simulink model "sys"  (R2020b)
settings: Solver=VariableStepAuto  StartTime=0.0  StopTime=10  RelTol=1e-3
values from neighbouring files (symbols this model uses):
  A = - 1 / (epsilon * Td)    (= -10)    [script.m]
  B = [ 1/(epsilon * Td) 0 ]    [script.m]
  C = kd / epsilon    (= 0.0001)    [script.m]
  D = [ -k-kd/epsilon kr ]    [script.m]
  stateBar = [ hBar; qBar; NBar ]    [script.m]
  uBar = 0    [script.m]
libraries: simulink x1
settings Model: Creator=thoma  LastModifiedBy=thoma

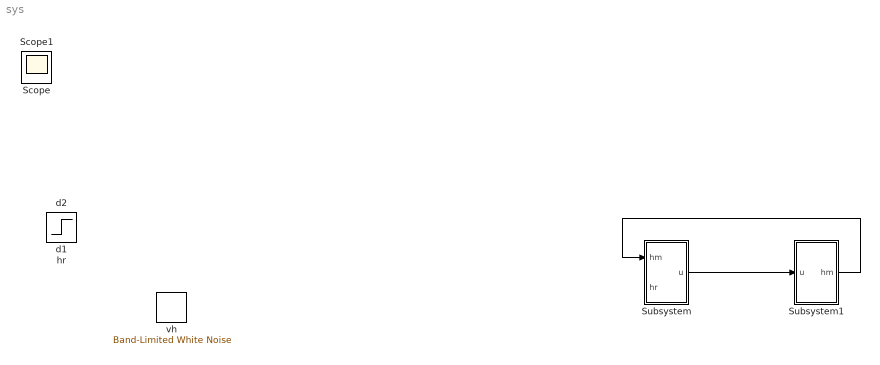
== system sys ==
  Subsystem : Subsystem
  Subsystem1 : Subsystem
  Scope : Scope
  Scope1 : Scope
  d1 : Step  IOType=siggen  After=0.2  SampleTime=0
  d2 : Step  IOType=siggen  Time=4  After=-1  SampleTime=0
  hr : Step  IOType=siggen  After=0  SampleTime=0
  vh : simulink/Sources/Band-Limited White Noise  IOType=siggen  Cov=1e-6  Ts=1e-2  seed=10
  wires:
  Subsystem/1(u) -> Subsystem1/1(u)
  Subsystem1/1(hm) -> Subsystem/1(hm)

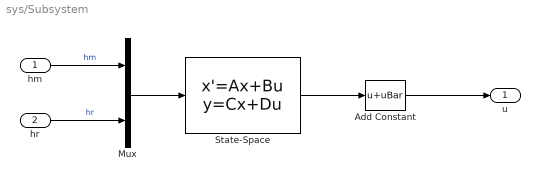
== system sys/Subsystem ==
  hm : Inport
  hr : Inport  Port=2
  Add Constant : Bias  Bias=uBar
  Mux : Mux  Inputs=2
  State-Space : StateSpace  A=A  B=B  C=C  D=D  InitialCondition=0
  u : Outport
  wires:
  Mux/1 -> State-Space/1
  State-Space/1 -> Add Constant/1
  Add Constant/1 -> u/1
  hm/1 -> Mux/1  "hm"
  hr/1 -> Mux/2  "hr"

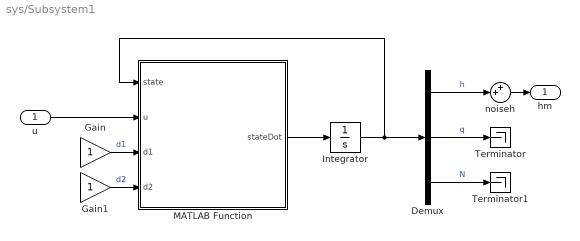
== system sys/Subsystem1 ==
  u : Inport
  Demux : Demux  Outputs=3
  Gain : Gain
  Gain1 : Gain
  Integrator : Integrator  InitialCondition=stateBar
  MATLAB Function : MATLAB Function  TreatAsAtomicUnit=on
  Terminator : Terminator
  Terminator1 : Terminator
  noiseh : Sum  Inputs=++|
  hm : Outport
  wires:
  Demux/3 -> Terminator1/1  "N"
  Demux/2 -> Terminator/1  "q"
  noiseh/1 -> hm/1
  Integrator/1 -> MATLAB Function/1(state), Demux/1
  Demux/1 -> noiseh/2  "h"
  MATLAB Function/1(stateDot) -> Integrator/1
  u/1 -> MATLAB Function/2(u)
  Gain/1 -> MATLAB Function/3(d1)  "d1"
  Gain1/1 -> MATLAB Function/4(d2)  "d2"

== matlab function sys/Subsystem1/MATLAB Function ==
  data: state input; u input; stateDot output; d1 input; d2 input
function stateDot = fcn(state, u, d1, d2)
h = state(1);
q = state(2);
N = state(3);

a = 1.0;
b = 2.5;
c = 0.1;
hBar = 0;
NBar = a/b;

hDot = q;
qDot = b*c*NBar*h - b*(1-c*hBar)*N + d2;
NDot = u + d1;
stateDot = [hDot; qDot; NDot];
